simulink model "Manimtim_Problem6"  (R2023b)
settings: Solver=VariableStepAuto  StartTime=0.0  StopTime=10.0  RelTol=1e-3
values from neighbouring files (symbols this model uses):
  G_den6 = [1 2 3 4 1]    [Manimtim_Problem5and6.m]
  G_num6 = [4 3 2 1]    [Manimtim_Problem5and6.m]
settings Model: Creator=John Kenneth  LastModifiedBy=John Kenneth

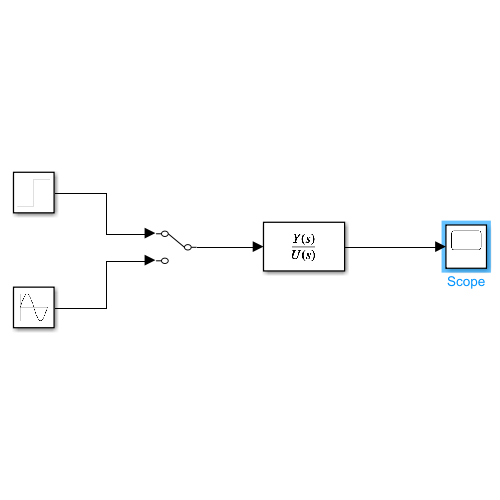
[thumbnail: Simulink's stored preview of the top-level diagram]
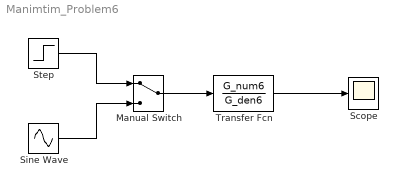
== system Manimtim_Problem6 ==
  Manual Switch : ManualSwitch
  Scope : Scope
  Sine Wave : Sin  SampleTime=0
  Step : Step  Time=0  SampleTime=0
  Transfer Fcn : TransferFcn  Numerator=G_num6  Denominator=G_den6
  wires:
  Step/1 -> Manual Switch/1
  Sine Wave/1 -> Manual Switch/2
  Manual Switch/1 -> Transfer Fcn/1
  Transfer Fcn/1 -> Scope/1
